simulink library "kfgpPrediction"  (R2020a)
settings: Solver=VariableStepAuto  StartTime=0.0  StopTime=10.0  RelTol=1e-3
values from neighbouring files (symbols this model uses):
  Amat = block.DialogPrm(1).Data    [altOptMPC_level2SFunc.m]    (also in kfgpPrediction_init.m = kron(eye(nAlt),F))
  Hmat = block.DialogPrm(3).Data    [altOptMPC_level2SFunc.m]    (also in kfgpPrediction_init.m = kron(eye(nAlt),H))
  Ks12 = block.DialogPrm(6).Data    [altOptMPC_level2SFunc.m]    (also in kfgpPrediction_init.m = sqrtm(Ks); kfgp_init.m = sqrtm(Ks))
  Qmat = block.DialogPrm(2).Data    [altOptMPC_level2SFunc.m]    (also in kfgpPrediction_init.m = kron(eye(nAlt),Q))
  Rmat = block.DialogPrm(4).Data    [altOptMPC_level2SFunc.m]    (also in kfgpPrediction_init.m = R)
  s0 = zeros(length(sigma0),1)    [kfgpPrediction_init.m]    (also in kfgp_init.m)
  sigma0 = removeEPS(lyap(F,G*G'),nRound)    [initializeKFGPForSquaredExponentialKernel.m]    (also in kfgpPrediction_init.m = kron(eye(nAlt),lyap(F,G*G')); kfgp_init.m = kron(eye(nAlt),lyap(F,G*G')))
settings Model: Creator=Ayaz  LastModifiedBy=Ayaz

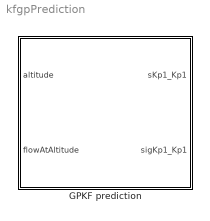
== system kfgpPrediction ==
  GPKF prediction : Subsystem  mask{gpkfTimeStep=1, timeScale=22*60, spatialScale=220, covAmp=1, xMeasure=100:100:1000, noiseVar=0.01, hTau='exponential', powerLawParams=[3.77 0.14]}
      mask prompts: gpkfTimeStep "Time step [s]"; timeScale "Temporal length scale [s]"; spatialScale "Altitude lenght scale [m]"; covAmp "Altitude covariance amplitude [-]"; xMeasure "Discreted altitudes measurement space [m]"; noiseVar "Noise variance [m^2/s^2]"; hTau "Temporal kernel"; powerLawParams "Power law parameters, mZ = a*z^b"
      mask init:
      | [Amat,Qmat,Hmat,Rmat,Ks,Ks12,s0,sigma0] = kfgp_init(xMeasure,covAmp,...
      |     spatialScale,noiseVar,hTau,gpkfTimeStep,timeScale);

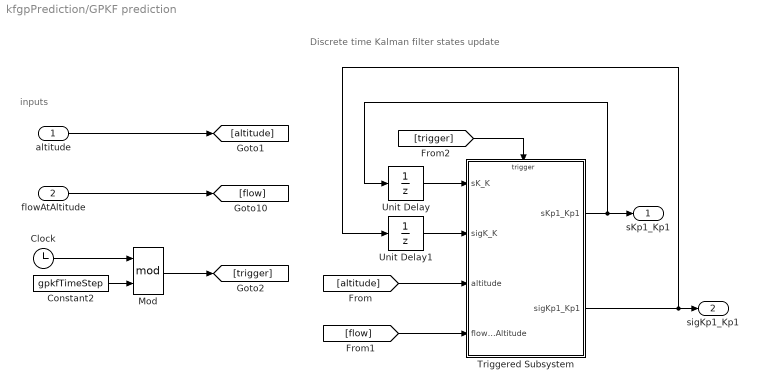
== system kfgpPrediction/GPKF prediction ==
  note: Discrete time Kalman filter states update
  note: inputs
  altitude : Inport
  flowAtAltitude : Inport  Port=2
  Clock : Clock
  Constant2 : Constant  Value=gpkfTimeStep  VectorParams1D=off
  Mod : Math  Operator=mod  SaturateOnIntegerOverflow=on
  Triggered Subsystem : Subsystem  TreatAsAtomicUnit=on
  Unit Delay : UnitDelay  InitialCondition=s0  SampleTime=-1  HasFrameUpgradeWarning=on
  Unit Delay1 : UnitDelay  InitialCondition=sigma0  SampleTime=-1  HasFrameUpgradeWarning=on
  sKp1_Kp1 : Outport
  sigKp1_Kp1 : Outport  Port=2
  wires:
  altitude/1 -> [altitude]
  flowAtAltitude/1 -> [flow]
  Unit Delay/1 -> Triggered Subsystem/1(sK_K)
  Unit Delay1/1 -> Triggered Subsystem/2(sigK_K)
  Triggered Subsystem/2(sigKp1_Kp1) -> sigKp1_Kp1/1, Unit Delay1/1
  [altitude] -> Triggered Subsystem/3(altitude)
  [flow] -> Triggered Subsystem/4(flowAtAltitude)
  Clock/1 -> Mod/1
  Constant2/1 -> Mod/2
  Mod/1 -> [trigger]
  [trigger] -> Triggered Subsystem/Trigger
  Triggered Subsystem/1(sKp1_Kp1) -> sKp1_Kp1/1, Unit Delay/1

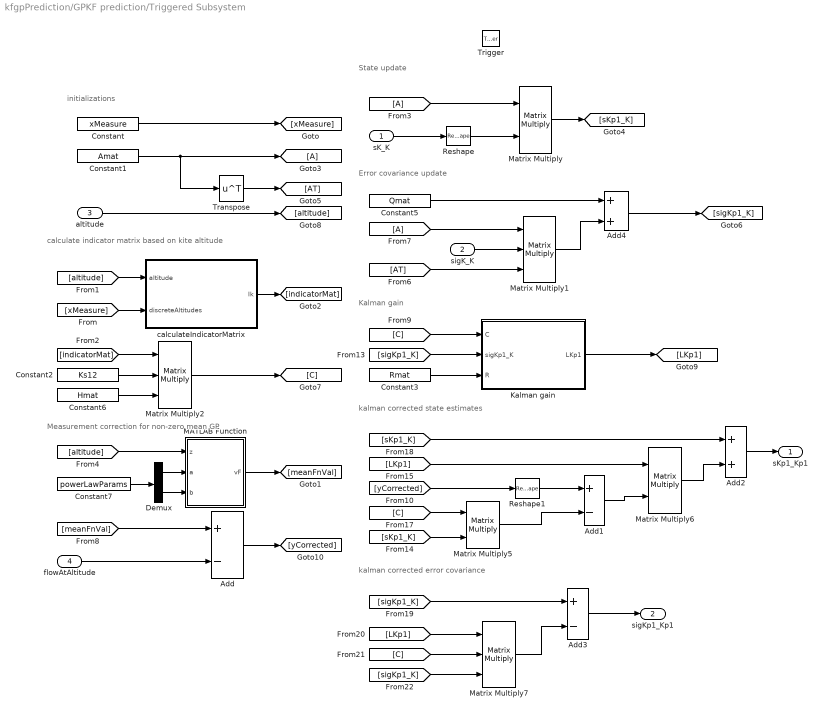
== system kfgpPrediction/GPKF prediction/Triggered Subsystem ==
  note: calculate indicator matrix based on kite altitude
  note: initializations
  note: Error covariance update
  note: Measurement correction for non-zero mean GP
  note: Kalman gain
  note: kalman corrected error covariance
  note: kalman corrected state estimates
  note: State update
  sK_K : Inport
  sigK_K : Inport  Port=2
  altitude : Inport  Port=3
  flowAtAltitude : Inport  Port=4
  Trigger : TriggerPort  VariantControl=Variant
  Add : Sum  Inputs=+-
  Add1 : Sum  Inputs=+-
  Add2 : Sum
  Add3 : Sum  Inputs=+-
  Add4 : Sum
  Constant : Constant  Value=xMeasure  VectorParams1D=off
  Constant1 : Constant  Value=Amat  VectorParams1D=off
  Constant2 : Constant  Value=Ks12  VectorParams1D=off
  Constant3 : Constant  Value=Rmat  VectorParams1D=off
  Constant5 : Constant  Value=Qmat  VectorParams1D=off
  Constant6 : Constant  Value=Hmat  VectorParams1D=off
  Constant7 : Constant  Value=powerLawParams
  Demux : Demux  Outputs=2
  Kalman gain : MATLAB Function  TreatAsAtomicUnit=on
  MATLAB Function : MATLAB Function  TreatAsAtomicUnit=on
  Matrix Multiply : Product  Multiplication=Matrix(*)
  Matrix Multiply1 : Product  Inputs=3  Multiplication=Matrix(*)
  Matrix Multiply2 : Product  Inputs=3  Multiplication=Matrix(*)
  Matrix Multiply5 : Product  Multiplication=Matrix(*)
  Matrix Multiply6 : Product  Multiplication=Matrix(*)
  Matrix Multiply7 : Product  Inputs=3  Multiplication=Matrix(*)
  Reshape : Reshape  OutputDimensionality=Column vector (2-D)
  Reshape1 : Reshape  OutputDimensionality=Column vector (2-D)
  Transpose : Math  Operator=transpose  SaturateOnIntegerOverflow=on
  calculateIndicatorMatrix : MATLAB Function  TreatAsAtomicUnit=on
  sKp1_Kp1 : Outport
  sigKp1_Kp1 : Outport  Port=2
  wires:
  [C] -> Matrix Multiply5/1
  [LKp1] -> Matrix Multiply6/1
  Matrix Multiply7/1 -> Add3/2
  Add2/1 -> sKp1_Kp1/1
  [sKp1_K] -> Matrix Multiply5/2
  [C] -> Matrix Multiply7/2
  sigK_K/1 -> Matrix Multiply1/2
  [sigKp1_K] -> Add3/1
  Matrix Multiply6/1 -> Add2/2
  [sigKp1_K] -> Matrix Multiply7/3
  [A] -> Matrix Multiply/1
  flowAtAltitude/1 -> Add/2
  [sKp1_K] -> Add2/1
  Matrix Multiply/1 -> [sKp1_K]
  [A] -> Matrix Multiply1/1
  Add3/1 -> sigKp1_Kp1/1
  [AT] -> Matrix Multiply1/3
  Matrix Multiply5/1 -> Add1/2
  [LKp1] -> Matrix Multiply7/1
  Constant3/1 -> Kalman gain/3(R)
  Add1/1 -> Matrix Multiply6/2
  sK_K/1 -> Reshape/1
  Transpose/1 -> [AT]
  Constant/1 -> [xMeasure]
  Constant1/1 -> Transpose/1, [A]
  [xMeasure] -> calculateIndicatorMatrix/2(discreteAltitudes)
  calculateIndicatorMatrix/1(Ik) -> [indicatorMat]
  altitude/1 -> [altitude]
  [C] -> Kalman gain/1(C)
  [sigKp1_K] -> Kalman gain/2(sigKp1_K)
  Kalman gain/1(LKp1) -> [LKp1]
  Reshape/1 -> Matrix Multiply/2
  Reshape1/1 -> Add1/1
  MATLAB Function/1(vF) -> [meanFnVal]
  [altitude] -> calculateIndicatorMatrix/1(altitude)
  [altitude] -> MATLAB Function/1(z)
  [meanFnVal] -> Add/1
  Add/1 -> [yCorrected]
  [yCorrected] -> Reshape1/1
  Constant5/1 -> Add4/1
  Matrix Multiply1/1 -> Add4/2
  Add4/1 -> [sigKp1_K]
  Matrix Multiply2/1 -> [C]
  Constant2/1 -> Matrix Multiply2/2
  [indicatorMat] -> Matrix Multiply2/1
  Constant6/1 -> Matrix Multiply2/3
  Demux/1 -> MATLAB Function/2(a)
  Demux/2 -> MATLAB Function/3(b)
  Constant7/1 -> Demux/1

== matlab function kfgpPrediction/GPKF prediction/Triggered Subsystem/calculateIndicatorMatrix ==
  data: altitude input; Ik output; discreteAltitudes input
function Ik = fcn(altitude,discreteAltitudes)
Ik = calculateIndicatorMat(altitude,discreteAltitudes);
end

== matlab function kfgpPrediction/GPKF prediction/Triggered Subsystem/MATLAB Function ==
  data: z input; vF output; a input; b input
function vF = fcn(z,a,b)

vF = powerLaw(z,a,b);

end

== matlab function kfgpPrediction/GPKF prediction/Triggered Subsystem/Kalman gain ==
  data: C input; LKp1 output; sigKp1_K input; R input
function LKp1 = fcn(C,sigKp1_K,R)

LKp1 = calculateKalmanGain(C,sigKp1_K,R);

end
